simulink model "Simulink_vector"  (R2017b)
settings: Solver=ode23t  StartTime=0.0  StopTime=5  RelTol=1e-3
values from neighbouring files (symbols this model uses):
  Cf = 400e-6    (= 0.0004)    [Parametros_Vector.m]
  Ks = 1/3*[-1 0 1;1 -1 0;0 1 -1]    [Parametros_Vector.m]
  Lf = 800e-6    (= 0.0008)    [Parametros_Vector.m]
  Lload = 2e-3    (= 0.002)    [Parametros_Vector.m]
  Rload = 50    [Parametros_Vector.m]
  Tz = 1/fz    (= 0.000333333333333)    [Parametros_Vector.m]
  V_ref = (2/3)*a*Vdc    (= 160)    [Parametros_Vector.m]
  Vdc = 400    [Parametros_Vector.m]
  w = 2*pi*60    (= 376.991118431)    [Parametros_Vector.m]
settings Model: Creator=USUARIO  LastModifiedBy=USUARIO

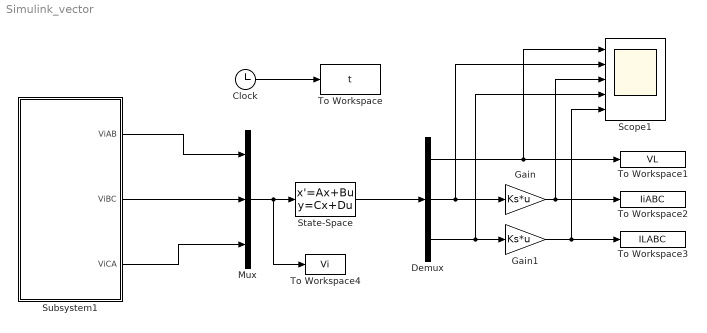
== system Simulink_vector ==
  Clock : Clock
  Demux : Demux  Outputs=3
  Gain : Gain  Gain=Ks*u
  Gain1 : Gain  Gain=Ks*u
  Mux : Mux  Inputs=3
  Scope1 : Scope  NumInputPorts=5
  State-Space : StateSpace  A=[zeros(3,3) eye(3)/(3*Cf) -eye(3)/(3*Cf); -eye(3)/Lf zeros(3,3) zeros(3,3);eye(3,3)/Lload zeros(3,3) -eye(3)*Rload/Lload]  B=[zeros(3,3); eye(3)/Lf; zeros(3,3)]  C=[eye(9)]  D=[zeros(9,3)]  InitialCondition=0
  Subsystem1 : Subsystem
  To Workspace : ToWorkspace  VariableName=t  SampleTime=-1
  To Workspace1 : ToWorkspace  VariableName=VL  SampleTime=-1
  To Workspace2 : ToWorkspace  VariableName=IiABC  SampleTime=-1
  To Workspace3 : ToWorkspace  VariableName=ILABC  SampleTime=-1
  To Workspace4 : ToWorkspace  VariableName=Vi  SampleTime=-1
  wires:
  Subsystem1/3(ViCA) -> Mux/3
  Subsystem1/2(ViBC) -> Mux/2
  Subsystem1/1(ViAB) -> Mux/1
  State-Space/1 -> Demux/1
  Demux/2 -> Scope1/2, Gain/1
  Clock/1 -> To Workspace/1
  Gain/1 -> Scope1/3, To Workspace2/1
  Demux/3 -> Gain1/1, Scope1/4
  Demux/1 -> Scope1/1, To Workspace1/1
  Mux/1 -> To Workspace4/1, State-Space/1
  Gain1/1 -> Scope1/5, To Workspace3/1

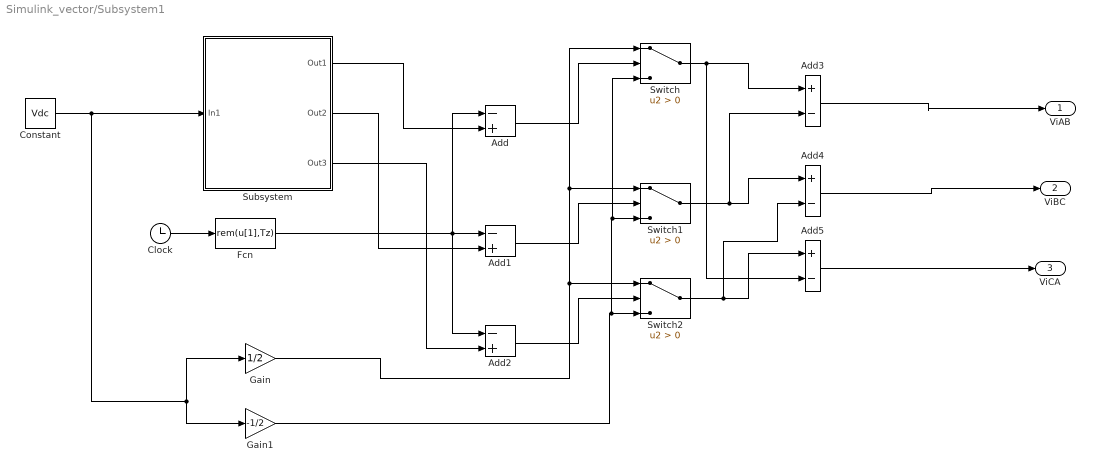
== system Simulink_vector/Subsystem1 ==
  Add : Sum  Inputs=-+
  Add1 : Sum  Inputs=-+
  Add2 : Sum  Inputs=-+
  Add3 : Sum  Inputs=+-
  Add4 : Sum  Inputs=+-
  Add5 : Sum  Inputs=+-
  Clock : Clock
  Constant : Constant  Value=Vdc
  Fcn : Fcn  Expr=rem(u[1],Tz)
  Gain : Gain  Gain=1/2
  Gain1 : Gain  Gain=-1/2
  Subsystem : Subsystem
  Switch : Switch  Criteria=u2 > Threshold
  Switch1 : Switch  Criteria=u2 > Threshold
  Switch2 : Switch  Criteria=u2 > Threshold
  ViAB : Outport
  ViBC : Outport  Port=2
  ViCA : Outport  Port=3
  wires:
  Switch1/1 -> Add3/2, Add4/1
  Switch2/1 -> Add4/2, Add5/1
  Subsystem/1(Out1) -> Add/2
  Subsystem/2(Out2) -> Add1/2
  Subsystem/3(Out3) -> Add2/2
  Fcn/1 -> Add/1, Add2/1, Add1/1
  Add3/1 -> ViAB/1
  Add4/1 -> ViBC/1
  Constant/1 -> Gain1/1, Gain/1, Subsystem/1(In1)
  Gain1/1 -> Switch/3, Switch1/3, Switch2/3
  Clock/1 -> Fcn/1
  Add1/1 -> Switch1/2
  Add5/1 -> ViCA/1
  Switch/1 -> Add5/2, Add3/1
  Gain/1 -> Switch2/1, Switch1/1, Switch/1
  Add/1 -> Switch/2
  Add2/1 -> Switch2/2

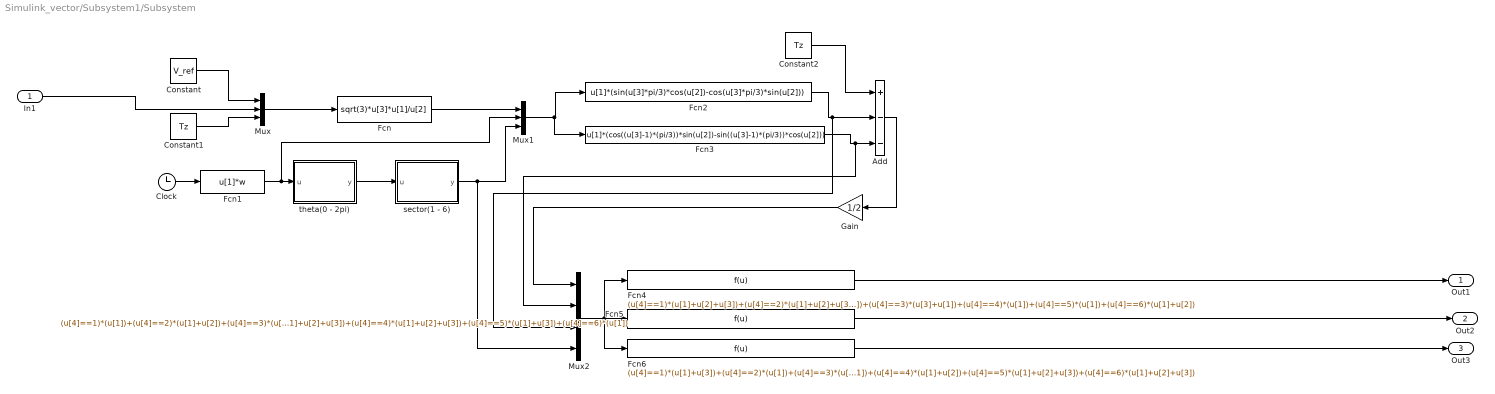
== system Simulink_vector/Subsystem1/Subsystem ==
  In1 : Inport
  Add : Sum  Inputs=+--
  Clock : Clock
  Constant : Constant  Value=V_ref
  Constant1 : Constant  Value=Tz
  Constant2 : Constant  Value=Tz
  Fcn : Fcn  Expr=sqrt(3)*u[3]*u[1]/u[2]
  Fcn1 : Fcn  Expr=u[1]*w
  Fcn2 : Fcn  Expr=u[1]*(sin(u[3]*pi/3)*cos(u[2])-cos(u[3]*pi/3)*sin(u[2]))
  Fcn3 : Fcn  Expr=u[1]*(cos((u[3]-1)*(pi/3))*sin(u[2])-sin((u[3]-1)*(pi/3))*cos(u[2]))
  Fcn4 : Fcn  Expr=(u[4]==1)*(u[1]+u[2]+u[3])+(u[4]==2)*(u[1]+u[2]+u[3])+(u[4]==3)*(u[3]+u[1])+(u[4]==4)*(u[1])+(u[4]==5)*(u[1])+(u[4]==6)*(u[1]+u[2])
  Fcn5 : Fcn  Expr=(u[4]==1)*(u[1])+(u[4]==2)*(u[1]+u[2])+(u[4]==3)*(u[1]+u[2]+u[3])+(u[4]==4)*(u[1]+u[2]+u[3])+(u[4]==5)*(u[1]+u[3])+(u[4]==6)*(u[1])
  Fcn6 : Fcn  Expr=(u[4]==1)*(u[1]+u[3])+(u[4]==2)*(u[1])+(u[4]==3)*(u[1])+(u[4]==4)*(u[1]+u[2])+(u[4]==5)*(u[1]+u[2]+u[3])+(u[4]==6)*(u[1]+u[2]+u[3])
  Gain : Gain  Gain=1/2
  Mux : Mux  Inputs=3
  Mux1 : Mux  Inputs=3
  Mux2 : Mux
  sector(1 - 6) : MATLAB Function  TreatAsAtomicUnit=on
  theta(0 - 2pi) : MATLAB Function  TreatAsAtomicUnit=on
  Out1 : Outport
  Out2 : Outport  Port=2
  Out3 : Outport  Port=3
  wires:
  theta(0 - 2pi)/1(y) -> sector(1 - 6)/1(u)
  Fcn1/1 -> Mux1/2, theta(0 - 2pi)/1(u)
  Clock/1 -> Fcn1/1
  sector(1 - 6)/1(y) -> Mux2/4, Mux1/3
  Constant/1 -> Mux/1
  Fcn/1 -> Mux1/1
  Gain/1 -> Mux2/1
  Constant2/1 -> Add/1
  Fcn6/1 -> Out3/1
  Fcn4/1 -> Out1/1
  Add/1 -> Gain/1
  Fcn3/1 -> Mux2/2, Add/3
  Mux2/1 -> Fcn6/1, Fcn5/1, Fcn4/1
  Mux/1 -> Fcn/1
  Fcn5/1 -> Out2/1
  Mux1/1 -> Fcn3/1, Fcn2/1
  Fcn2/1 -> Mux2/3, Add/2
  Constant1/1 -> Mux/3
  In1/1 -> Mux/2

== matlab function Simulink_vector/Subsystem1/Subsystem/sector(1 - 6) ==
  data: u input; y output
function y = fcn(u)
%#codegen

y = 1+ fix(u/(pi/3+1.e-30));

== matlab function Simulink_vector/Subsystem1/Subsystem/theta(0 - 2pi) ==
  data: u input; y output
function y = fcn(u)
%#codegen

y = mod(u,2*pi);
